simulink model "foc_mtpa_fw_test_2"  (R2015a)
settings: Solver=ode4  StartTime=0.0  StopTime=8  FixedStep=2e-5  RelTol=1e-3
libraries: simulink x2
settings Model: Creator=user  LastModifiedBy=user

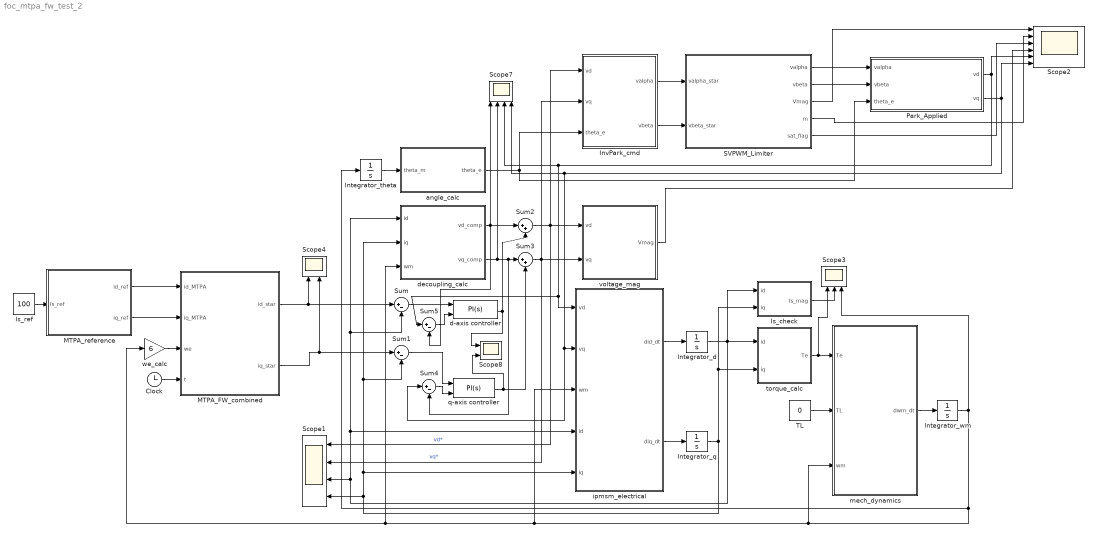
== system foc_mtpa_fw_test_2 ==
  Clock : Clock
  Integrator_d : Integrator
  Integrator_q : Integrator
  Integrator_theta : Integrator
  Integrator_wm : Integrator
  InvPark_cmd : MATLAB Function  TreatAsAtomicUnit=on
  Is_check : MATLAB Function  TreatAsAtomicUnit=on
  Is_ref : Constant  Value=100
  MTPA_FW_combined : MATLAB Function  TreatAsAtomicUnit=on
  MTPA_reference : MATLAB Function  TreatAsAtomicUnit=on
  Park_Applied : MATLAB Function  TreatAsAtomicUnit=on
  SVPWM_Limiter : MATLAB Function  TreatAsAtomicUnit=on
  Scope1 : Scope  NumInputPorts=4
      settings: YMin=-5~-5~-5~-5  YMax=5~5~5~5  SaveName=ScopeData2
  Scope2 : Scope  NumInputPorts=6
      settings: YMin=-5~-5~-5~-5~-5~-5  YMax=5~5~5~5~5~5
  Scope3 : Scope  NumInputPorts=3
      settings: YMin=-5~-5~-5  YMax=5~5~5
  Scope4 : Scope  NumInputPorts=2
      settings: YMin=-5~-5  YMax=5~5  SaveName=ScopeData3  ScrollMode=on
  Scope7 : Scope  NumInputPorts=4
      settings: YMin=-5~-5~-5~-5  YMax=5~5~5~5  SaveName=ScopeData6
  Scope8 : Scope  NumInputPorts=2
      settings: YMin=-5~-5  YMax=5~5  SaveName=ScopeData7
  Sum{,1,4..5} (4 alike) : Sum  Inputs=|+-
  Sum2 : Sum  Inputs=|++
  Sum3 : Sum  Inputs=|++
  TL : Constant  Value=0
  angle_calc : MATLAB Function  TreatAsAtomicUnit=on
  d-axis controller : simulink/Continuous/PID Controller  Controller=PI  TimeDomain=Continuous-time  SampleTime=-1  IntegratorMethod=Forward Euler  FilterMethod=Forward Euler  Form=Parallel  UseFilter=on  ControllerParametersSource=internal  P=0.2827  I=16.6504  D=0  N=100  InitialConditionSource=internal  InitialConditionForIntegrator=0  InitialConditionForFilter=0  ExternalReset=none  LimitOutput=on  UpperSaturationLimit=207.85  LowerSaturationLimit=-207.85  LinearizeAsGain=on  AntiWindupMode=back-calculation  Kb=16.6504  TrackingMode=on  Kt=83.252  PParamMin=[]  PParamMax=[]  IParamMin=[]  IParamMax=[]  DParamMin=[]  DParamMax=[]  NParamMin=[]  NParamMax=[]  KbParamMin=[]  KbParamMax=[]  KtParamMin=[]  KtParamMax=[]  POutMin=[]  POutMax=[]  IOutMin=[]  IOutMax=[]  DOutMin=[]  DOutMax=[]  NOutMin=[]  NOutMax=[]  KbOutMin=[]  KbOutMax=[]  KtOutMin=[]  KtOutMax=[]  IntegratorOutMin=[]  IntegratorOutMax=[]  FilterOutMin=[]  FilterOutMax=[]  SumOutMin=[]  SumOutMax=[]  SumI1OutMin=[]  SumI1OutMax=[]  SumI2OutMin=[]  SumI2OutMax=[]  SumI3OutMin=[]  SumI3OutMax=[]  SumDOutMin=[]  SumDOutMax=[]  SaturationOutMin=[]  SaturationOutMax=[]  IntegratorContinuousStateAttributes=''  IntegratorStateMustResolveToSignalObject=off  IntegratorRTWStateStorageClass=Auto  FilterContinuousStateAttributes=''  FilterStateMustResolveToSignalObject=off  FilterRTWStateStorageClass=Auto  DifferentiatorICPrevScaledInput=0  DifferentiatorOutMin=[]  DifferentiatorOutMax=[]
  decoupling_calc : MATLAB Function  TreatAsAtomicUnit=on
  ipmsm_electrical : MATLAB Function  TreatAsAtomicUnit=on
  mech_dynamics : MATLAB Function  TreatAsAtomicUnit=on
  q-axis controller : simulink/Continuous/PID Controller  Controller=PI  TimeDomain=Continuous-time  SampleTime=-1  IntegratorMethod=Forward Euler  FilterMethod=Forward Euler  Form=Parallel  UseFilter=on  ControllerParametersSource=internal  P=0.8011  I=16.6504  D=0  N=100  InitialConditionSource=internal  InitialConditionForIntegrator=0  InitialConditionForFilter=0  ExternalReset=none  LimitOutput=on  UpperSaturationLimit=207.85  LowerSaturationLimit=-207.85  LinearizeAsGain=on  AntiWindupMode=back-calculation  Kb=16.6504  TrackingMode=on  Kt=83.252  PParamMin=[]  PParamMax=[]  IParamMin=[]  IParamMax=[]  DParamMin=[]  DParamMax=[]  NParamMin=[]  NParamMax=[]  KbParamMin=[]  KbParamMax=[]  KtParamMin=[]  KtParamMax=[]  POutMin=[]  POutMax=[]  IOutMin=[]  IOutMax=[]  DOutMin=[]  DOutMax=[]  NOutMin=[]  NOutMax=[]  KbOutMin=[]  KbOutMax=[]  KtOutMin=[]  KtOutMax=[]  IntegratorOutMin=[]  IntegratorOutMax=[]  FilterOutMin=[]  FilterOutMax=[]  SumOutMin=[]  SumOutMax=[]  SumI1OutMin=[]  SumI1OutMax=[]  SumI2OutMin=[]  SumI2OutMax=[]  SumI3OutMin=[]  SumI3OutMax=[]  SumDOutMin=[]  SumDOutMax=[]  SaturationOutMin=[]  SaturationOutMax=[]  IntegratorContinuousStateAttributes=''  IntegratorStateMustResolveToSignalObject=off  IntegratorRTWStateStorageClass=Auto  FilterContinuousStateAttributes=''  FilterStateMustResolveToSignalObject=off  FilterRTWStateStorageClass=Auto  DifferentiatorICPrevScaledInput=0  DifferentiatorOutMin=[]  DifferentiatorOutMax=[]
  torque_calc : MATLAB Function  TreatAsAtomicUnit=on
  voltage_mag : MATLAB Function  TreatAsAtomicUnit=on
  we_calc : Gain  Gain=6
  wires:
  Sum/1 -> d-axis controller/1
  Integrator_q/1 -> decoupling_calc/2(iq), Sum1/2, ipmsm_electrical/5(iq), Scope1/4, Is_check/2(iq), torque_calc/2(iq)
  Sum1/1 -> q-axis controller/1
  ipmsm_electrical/2(diq_dt) -> Integrator_q/1
  ipmsm_electrical/1(did_dt) -> Integrator_d/1
  Integrator_d/1 -> Is_check/1(id), torque_calc/1(id), decoupling_calc/1(id), Sum/2, ipmsm_electrical/4(id), Scope1/3
  Integrator_wm/1 -> mech_dynamics/3(wm), we_calc/1, decoupling_calc/3(wm), ipmsm_electrical/3(wm), Integrator_theta/1, Scope3/3
  decoupling_calc/1(vd_comp) -> Scope7/1, Sum5/2, Sum2/1
  d-axis controller/1 -> Sum2/2, Scope8/1
  decoupling_calc/2(vq_comp) -> Scope7/2, Sum4/2, Sum3/1
  q-axis controller/1 -> Scope8/2, Sum3/2
  Sum3/1 -> InvPark_cmd/2(vq), voltage_mag/2(vq), Scope1/2  "vq*"
  Sum2/1 -> InvPark_cmd/1(vd), voltage_mag/1(vd), Scope1/1  "vd*"
  torque_calc/1(Te) -> mech_dynamics/1(Te), Scope3/1
  TL/1 -> mech_dynamics/2(TL)
  mech_dynamics/1(dwm_dt) -> Integrator_wm/1
  Integrator_theta/1 -> angle_calc/1(theta_m)
  angle_calc/1(theta_e) -> InvPark_cmd/3(theta_e), Park_Applied/3(theta_e)
  InvPark_cmd/1(valpha) -> SVPWM_Limiter/1(valpha_star)
  InvPark_cmd/2(vbeta) -> SVPWM_Limiter/2(vbeta_star)
  SVPWM_Limiter/1(valpha) -> Park_Applied/1(valpha)
  SVPWM_Limiter/2(vbeta) -> Park_Applied/2(vbeta)
  SVPWM_Limiter/4(m) -> Scope2/2
  SVPWM_Limiter/3(Vmag) -> Scope2/1
  SVPWM_Limiter/5(sat_flag) -> Scope2/3
  voltage_mag/1(Vmag) -> Scope2/4
  Park_Applied/1(vd) -> Scope7/3, ipmsm_electrical/1(vd), Sum5/1, Scope2/5
  Park_Applied/2(vq) -> Scope7/4, Sum4/1, ipmsm_electrical/2(vq), Scope2/6
  Is_ref/1 -> MTPA_reference/1(Is_ref)
  Is_check/1(Is_mag) -> Scope3/2
  Sum5/1 -> d-axis controller/2
  Sum4/1 -> q-axis controller/2
  MTPA_reference/1(id_ref) -> MTPA_FW_combined/1(id_MTPA)
  MTPA_reference/2(iq_ref) -> MTPA_FW_combined/2(iq_MTPA)
  we_calc/1 -> MTPA_FW_combined/3(we)
  Clock/1 -> MTPA_FW_combined/4(t)
  MTPA_FW_combined/1(id_star) -> Scope4/1, Sum/1
  MTPA_FW_combined/2(iq_star) -> Scope4/2, Sum1/1

== matlab function foc_mtpa_fw_test_2/decoupling_calc ==
  data: id input; vd_comp output; iq input; wm input; vq_comp output
function [vd_comp, vq_comp] = decoupling_calc(id, iq, wm)
% Feedforward decoupling terms for BMW i3 IPMSM

Ld       = 0.090e-3;
Lq       = 0.255e-3;
lambda_m = 0.0385;
p        = 6;

we = p*wm;

vd_comp = -we*Lq*iq;
vq_comp =  we*(Ld*id + lambda_m);

end

== matlab function foc_mtpa_fw_test_2/ipmsm_electrical ==
  data: vd input; did_dt output; vq input; wm input; id input; iq input; diq_dt output
function [did_dt, diq_dt] = ipmsm_electrical(vd, vq, wm, id, iq)
% BMW i3 IPMSM dq-axis electrical dynamics
% Units: V, rad/s, A, A/s

Rs       = 5.3e-3;    % Stator resistance, Ohm
Ld       = 0.090e-3;  % d-axis inductance, H
Lq       = 0.255e-3;  % q-axis inductance, H
lambda_m = 0.0385;    % PM flux linkage, Wb
p        = 6;         % Pole pairs

we = p*wm;             % electrical angular velocity, rad/s

did_dt = (vd - Rs*id + we*Lq*iq) / Ld;
diq_dt = (vq - Rs*iq - we*(Ld*id + lambda_m)) / Lq;

end

== matlab function foc_mtpa_fw_test_2/torque_calc ==
  data: id input; Te output; iq input
function Te = torque_calc(id, iq)
% BMW i3 electromagnetic torque
% Units: id, iq in A; Te in Nm

Ld       = 0.090e-3;
Lq       = 0.255e-3;
lambda_m = 0.0385;
p        = 6;

Te = (3/2) * p * (lambda_m*iq + (Ld - Lq)*id*iq);

end

== matlab function foc_mtpa_fw_test_2/mech_dynamics ==
  data: Te input; dwm_dt output; TL input; wm input
function dwm_dt = mech_dynamics(Te, TL, wm)
% BMW i3 mechanical dynamics
% Units: Te, TL in Nm; wm in rad/s; dwm_dt in rad/s^2

J = 0.06;    % ASSUMED
B = 0.001;   % ASSUMED

dwm_dt = (Te - TL - B*wm) / J;

end

== matlab function foc_mtpa_fw_test_2/angle_calc ==
  data: theta_m input; theta_e output
function theta_e = angle_calc(theta_m)
% Electrical angle from mechanical angle
p = 6;
theta_e = p*theta_m;
end

== matlab function foc_mtpa_fw_test_2/voltage_mag ==
  data: vd input; Vmag output; vq input
function Vmag = voltage_mag(vd, vq)
% Commanded voltage vector magnitude
Vmag = sqrt(vd^2 + vq^2);
end

== matlab function foc_mtpa_fw_test_2/InvPark_cmd ==
  data: vd input; valpha output; vq input; theta_e input; vbeta output
function [valpha, vbeta] = InvPark_cmd(vd, vq, theta_e)

valpha = vd*cos(theta_e) - vq*sin(theta_e);

vbeta = vd*sin(theta_e) + vq*cos(theta_e);

== matlab function foc_mtpa_fw_test_2/SVPWM_Limiter ==
  data: valpha_star input; valpha output; vbeta_star input; vbeta output; Vmag output; m output; sat_flag output
function [valpha, vbeta, Vmag, m, sat_flag] = SVPWM_Limiter(valpha_star, vbeta_star)

Vmax = 360/sqrt(3);

Vmag = sqrt(valpha_star^2 + vbeta_star^2);

m = Vmag/Vmax;

if Vmag <= Vmax
    valpha = valpha_star;
    vbeta = vbeta_star;
    sat_flag = 0;
else
    scale = Vmax/Vmag;
    valpha = valpha_star*scale;
    vbeta = vbeta_star*scale;
    sat_flag = 1;
end

== matlab function foc_mtpa_fw_test_2/Park_Applied ==
  data: valpha input; vbeta input; theta_e input; vd output; vq output
function [vd, vq] = Park_Applied(valpha, vbeta, theta_e)

vd = valpha*cos(theta_e) + vbeta*sin(theta_e);
vq = -valpha*sin(theta_e) + vbeta*cos(theta_e);

== matlab function foc_mtpa_fw_test_2/MTPA_reference ==
  data: Is_ref input; id_ref output; iq_ref output
function [id_ref, iq_ref] = MTPA_reference(Is_ref)

Ld = 0.090e-3;
Lq = 0.255e-3;
lambda_m = 0.0385;

DeltaL = Lq - Ld;

id_ref = (lambda_m - sqrt(lambda_m^2 + ...
          4*(DeltaL^2)*(Is_ref^2))) / (2*DeltaL);

iq_ref = sqrt(Is_ref^2 - id_ref^2);

== matlab function foc_mtpa_fw_test_2/MTPA_FW_combined ==
  data: id_MTPA input; id_star output; iq_star output; iq_MTPA input; we input; t input
function [id_star, iq_star] = MTPA_FW_combined(id_MTPA, iq_MTPA, we, t)
% Combines: FW id-target calculation, id rate limiting, and iq coupling
% into one atomic block. Replaces FW_reference, Cart2Polar, Polar2Cart,
% Is_mag_RateLimiter, Gamma_RateLimiter, and iq_star_calc.

persistent id_prev t_prev initialized
if isempty(initialized)
    id_prev = id_MTPA;
    t_prev = t;
    initialized = true;
end

Ld       = 0.090e-3;
Lq       = 0.255e-3;
lambda_m = 0.0385;
Is_max   = 430;
Vmax     = 207.85;
max_rate = 3000;   % A/s -- id slew rate, tune if needed

% --- Flux-weakening candidate id (voltage-ellipse boundary) ---
if abs(we) < 1e-6
    id_FW = id_MTPA;
else
    arg = (Vmax/we)^2 - (Lq*iq_MTPA)^2;
    arg = max(arg, 0);   % guard against infeasible demand (Region IV)
    id_FW = -lambda_m/Ld + (1/Ld)*sqrt(arg);
end

id_target = min(id_MTPA, id_FW);      % MTPA above base speed, FW below it
id_target = max(id_target, -Is_max);  % never exceed current limit alone

% --- Rate-limit id (manual, variable-step-safe) ---
dt = t - t_prev;
if dt <= 0
    dt = 1e-6;
end
max_step = max_rate*dt;
delta = max(min(id_target - id_prev, max_step), -max_step);
id_star = id_prev + delta;

id_prev = id_star;
t_prev  = t;

% --- Couple iq to the RATE-LIMITED id -- guarantees id^2+iq^2<=Is_max^2
% at every instant, eliminating the earlier transition discontinuity ---
iq_max_avail = sqrt(max(Is_max^2 - id_star^2, 0));
iq_star = min(iq_MTPA, iq_max_avail);

end

== matlab function foc_mtpa_fw_test_2/Is_check ==
  data: id input; Is_mag output; iq input
function Is_mag = Is_check(id, iq)
Is_mag = sqrt(id^2 + iq^2);
end
